simulink model "IDM_MOBIL"  (R2020a)
settings: Solver=VariableStepAuto  StartTime=0.0  StopTime=10.0  RelTol=1e-3
settings Model: Creator=Administrator  LastModifiedBy=Administrator

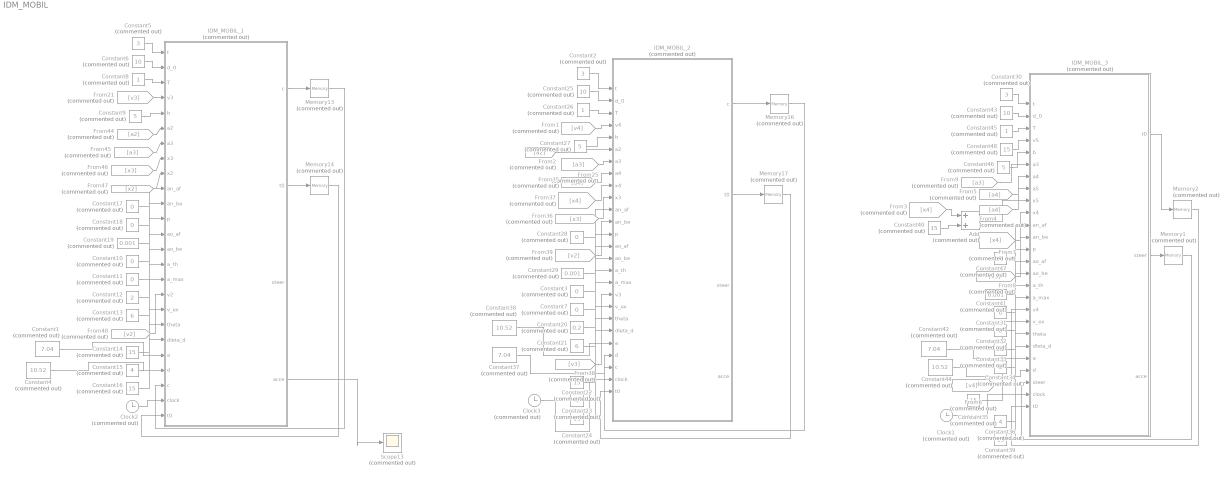
== system IDM_MOBIL ==
  Add : Sum  Commented=on
  Clock1 : Clock  Commented=on
  Clock2 : Clock  Commented=on
  Clock3 : Clock  Commented=on
  Constant1 : Constant  Commented=on  Value=7.04
  Constant{3,7,10..11,17..18,28,31..32,47} (10 alike) : Constant  Commented=on  Value=0
  Constant12 : Constant  Commented=on  Value=2
  Constant13 : Constant  Commented=on  Value=6
  Constant{14,16,22,24,35,39..40,48} (8 alike) : Constant  Commented=on  Value=15
  Constant15 : Constant  Commented=on  Value=4
  Constant19 : Constant  Commented=on  Value=0.001
  Constant2 : Constant  Commented=on  Value=3
  Constant20 : Constant  Commented=on  Value=0.2
  Constant21 : Constant  Commented=on  Value=6
  Constant23 : Constant  Commented=on  Value=4
  Constant25 : Constant  Commented=on  Value=10
  Constant26 : Constant  Commented=on
  Constant27 : Constant  Commented=on  Value=5
  Constant29 : Constant  Commented=on  Value=0.001
  Constant30 : Constant  Commented=on  Value=3
  Constant33 : Constant  Commented=on  Value=0.2
  Constant34 : Constant  Commented=on  Value=6
  Constant36 : Constant  Commented=on  Value=4
  Constant37 : Constant  Commented=on  Value=7.04
  Constant38 : Constant  Commented=on  Value=10.52
  Constant4 : Constant  Commented=on  Value=10.52
  Constant41 : Constant  Commented=on  Value=0.001
  Constant42 : Constant  Commented=on  Value=7.04
  Constant43 : Constant  Commented=on  Value=10
  Constant44 : Constant  Commented=on  Value=10.52
  Constant45 : Constant  Commented=on
  Constant46 : Constant  Commented=on  Value=5
  Constant5 : Constant  Commented=on  Value=3
  Constant6 : Constant  Commented=on  Value=10
  Constant8 : Constant  Commented=on
  Constant9 : Constant  Commented=on  Value=5
  From1 : From  Commented=on  GotoTag=v4  TagVisibility=global
  From2 : From  Commented=on  GotoTag=a2  TagVisibility=global
  From21 : From  Commented=on  GotoTag=v3  TagVisibility=global
  From25 : From  Commented=on  GotoTag=a3  TagVisibility=global
  From3 : From  Commented=on  GotoTag=x4  TagVisibility=global
  From35 : From  Commented=on  GotoTag=a4  TagVisibility=global
  From36 : From  Commented=on  GotoTag=x3  TagVisibility=global
  From37 : From  Commented=on  GotoTag=x4  TagVisibility=global
  From38 : From  Commented=on  GotoTag=v3  TagVisibility=global
  From39 : From  Commented=on  GotoTag=v2  TagVisibility=global
  From4 : From  Commented=on  GotoTag=a4  TagVisibility=global
  From44 : From  Commented=on  GotoTag=a2  TagVisibility=global
  From45 : From  Commented=on  GotoTag=a3  TagVisibility=global
  From46 : From  Commented=on  GotoTag=x3  TagVisibility=global
  From47 : From  Commented=on  GotoTag=x2  TagVisibility=global
  From48 : From  Commented=on  GotoTag=v2  TagVisibility=global
  From5 : From  Commented=on  GotoTag=a4  TagVisibility=global
  From6 : From  Commented=on  GotoTag=v4  TagVisibility=global
  From7 : From  Commented=on  GotoTag=x4  TagVisibility=global
  From8 : From  Commented=on  GotoTag=v3  TagVisibility=global
  From9 : From  Commented=on  GotoTag=a3  TagVisibility=global
  IDM_MOBIL_1 : MATLAB Function  Commented=on  TreatAsAtomicUnit=on
  IDM_MOBIL_2 : MATLAB Function  Commented=on  TreatAsAtomicUnit=on
  IDM_MOBIL_3 : MATLAB Function  Commented=on  TreatAsAtomicUnit=on
  Memory1 : Memory  Commented=on  InitialCondition=7.04
  Memory13 : Memory  Commented=on  InitialCondition=7.04
  Memory14 : Memory  Commented=on  InitialCondition=-3
  Memory16 : Memory  Commented=on  InitialCondition=10.52
  Memory17 : Memory  Commented=on  InitialCondition=-3
  Memory2 : Memory  Commented=on  InitialCondition=-3
  Scope13 : Scope  Commented=on
  wires:
  From48/1 -> IDM_MOBIL_1/17(v2)
  IDM_MOBIL_1/2(t0) -> Memory14/1
  Memory14/1 -> IDM_MOBIL_1/25("t0 ")
  Constant12/1 -> IDM_MOBIL_1/15(a_th)
  Memory13/1 -> IDM_MOBIL_1/23("c ")
  From47/1 -> IDM_MOBIL_1/9(x2)
  Constant15/1 -> IDM_MOBIL_1/19(theta)
  Constant10/1 -> IDM_MOBIL_1/13(ao_af)
  Constant16/1 -> IDM_MOBIL_1/20(dleta_d)
  Constant11/1 -> IDM_MOBIL_1/14(ao_be)
  Constant14/1 -> IDM_MOBIL_1/18(v_ex)
  From45/1 -> IDM_MOBIL_1/7(a3)
  Constant13/1 -> IDM_MOBIL_1/16(a_max)
  Constant5/1 -> IDM_MOBIL_1/1(t)
  From46/1 -> IDM_MOBIL_1/8(x3)
  Constant17/1 -> IDM_MOBIL_1/10(an_af)
  Constant19/1 -> IDM_MOBIL_1/12(p)
  Constant18/1 -> IDM_MOBIL_1/11(an_be)
  Clock2/1 -> IDM_MOBIL_1/24(clock)
  From44/1 -> IDM_MOBIL_1/6(a2)
  IDM_MOBIL_1/1(c) -> Memory13/1
  Constant4/1 -> IDM_MOBIL_1/22(d)
  Constant8/1 -> IDM_MOBIL_1/3(T)
  Constant1/1 -> IDM_MOBIL_1/21(a)
  IDM_MOBIL_1/4(acce) -> Scope13/1
  Constant6/1 -> IDM_MOBIL_1/2(d_0)
  From21/1 -> IDM_MOBIL_1/4(v3)
  Constant9/1 -> IDM_MOBIL_1/5(b)
  Constant21/1 -> IDM_MOBIL_2/17(a_max)
  Constant23/1 -> IDM_MOBIL_2/20(theta)
  Constant25/1 -> IDM_MOBIL_2/2(d_0)
  Constant24/1 -> IDM_MOBIL_2/21(dleta_d)
  Constant7/1 -> IDM_MOBIL_2/15(ao_be)
  IDM_MOBIL_2/1(c) -> Memory16/1
  IDM_MOBIL_2/2(t0) -> Memory17/1
  From2/1 -> IDM_MOBIL_2/6(a2)
  Constant37/1 -> IDM_MOBIL_2/23(d)
  Clock3/1 -> IDM_MOBIL_2/25(clock)
  Constant22/1 -> IDM_MOBIL_2/19(v_ex)
  Constant29/1 -> IDM_MOBIL_2/13(p)
  From38/1 -> IDM_MOBIL_2/18(v3)
  Memory17/1 -> IDM_MOBIL_2/26("t0 ")
  Constant20/1 -> IDM_MOBIL_2/16(a_th)
  Constant28/1 -> IDM_MOBIL_2/11(an_af)
  From25/1 -> IDM_MOBIL_2/7(a3)
  From37/1 -> IDM_MOBIL_2/9(x4)
  Constant3/1 -> IDM_MOBIL_2/14(ao_af)
  Constant38/1 -> IDM_MOBIL_2/22(a)
  Constant2/1 -> IDM_MOBIL_2/1(t)
  From39/1 -> IDM_MOBIL_2/12(an_be)
  From1/1 -> IDM_MOBIL_2/4(v4)
  Constant27/1 -> IDM_MOBIL_2/5(b)
  From36/1 -> IDM_MOBIL_2/10(x3)
  From35/1 -> IDM_MOBIL_2/8(a4)
  Constant26/1 -> IDM_MOBIL_2/3(T)
  Memory16/1 -> IDM_MOBIL_2/24("c ")
  IDM_MOBIL_3/1(t0) -> Memory2/1
  Constant47/1 -> IDM_MOBIL_3/11(an_af)
  Memory1/1 -> IDM_MOBIL_3/24("steer ")
  Constant36/1 -> IDM_MOBIL_3/20(theta)
  Memory2/1 -> IDM_MOBIL_3/26("t0 ")
  IDM_MOBIL_3/2(steer) -> Memory1/1
  From4/1 -> IDM_MOBIL_3/8(a5)
  Constant35/1 -> IDM_MOBIL_3/19(v_ex)
  Constant44/1 -> IDM_MOBIL_3/23(d)
  Constant34/1 -> IDM_MOBIL_3/17(a_max)
  Constant39/1 -> IDM_MOBIL_3/21(dleta_d)
  Constant31/1 -> IDM_MOBIL_3/14(ao_af)
  Constant42/1 -> IDM_MOBIL_3/22(a)
  From8/1 -> IDM_MOBIL_3/12(an_be)
  From6/1 -> IDM_MOBIL_3/18(v4)
  Constant46/1 -> IDM_MOBIL_3/5(b)
  From9/1 -> IDM_MOBIL_3/6(a3)
  From3/1 -> Add/1
  Constant48/1 -> IDM_MOBIL_3/4(v5)
  Constant30/1 -> IDM_MOBIL_3/1(t)
  From5/1 -> IDM_MOBIL_3/7(a4)
  Constant45/1 -> IDM_MOBIL_3/3(T)
  Constant32/1 -> IDM_MOBIL_3/15(ao_be)
  Clock1/1 -> IDM_MOBIL_3/25(clock)
  Constant43/1 -> IDM_MOBIL_3/2(d_0)
  Constant33/1 -> IDM_MOBIL_3/16(a_th)
  Constant41/1 -> IDM_MOBIL_3/13(p)
  From7/1 -> IDM_MOBIL_3/10(x4)
  Add/1 -> IDM_MOBIL_3/9(x5)
  Constant40/1 -> Add/2

== matlab function IDM_MOBIL/IDM_MOBIL_3 ==
  data: t0 output; t input; d_0 input; steer output; T input; v5 input; b input; a3 input; a4 input; a5 input; x5 input; x4 input; an_af input; an_be input; p input; ao_af input; ao_be input; a_th input; a_max input; v4 input; v_ex input; theta input; dleta_d input; acce output; a input; d input; steer input; clock input; t0 input
function [t0,steer,acce] = fcn(t,d_0,T,v5,b,a3,a4,a5,x5,x4,an_af,an_be,p,ao_af,ao_be,a_th,a_max,v4,v_ex,theta,dleta_d,a,d,steer,clock,t0)
delta_t = 3.5;
ac_be = a4;
vc_af = v4 + a4*t;
dleta_v = v5-v4;
dleta_cv_af = v5+a5*t-vc_af;
an_af = an_af+an_be+a3*t;
dleta_cd = x5+v5*t+0.5*a5*t^2-(x4+v4*t+0.5*a4*t^2);
dc_ex = d_0+T*vc_af+(vc_af*dleta_cv_af/(2*sqrt(a_max*b)));
ac_af = a_max*(1-(vc_af/v_ex)^theta-(dc_ex/dleta_cd)^2);
d_ex = d_0+T*v4+(v4*dleta_v/(2*sqrt(a_max*b)));
if clock-t0 > delta_t
    if ac_af-ac_be+p*(an_af-an_be+ao_af-ao_be) >= a_th
        if steer==a
            steer=d;
            acce = 0;
            t0=clock;
        else
            steer=a;
            acce = 0;
            t0=clock;
        end
    else
        steer=steer;
        acce = a_max*(1-(v4/v_ex)^theta-(d_ex/dleta_d)^2);
    end
else
    steer=steer;
    acce = 0;
    %acce = a_max*(1-(v4/v_ex)^theta-(d_ex/dleta_d)^2);
end

== matlab function IDM_MOBIL/IDM_MOBIL_1 ==
  data: c output; t0 output; t input; d_0 input; steer output; T input; v3 input; b input; a2 input; a3 input; x3 input; x2 input; an_af input; an_be input; p input; ao_af input; ao_be input; a_th input; a_max input; v2 input; v_ex input; theta input; dleta_d input; acce output; a input; d input; c input; clock input; t0 input
function [c,t0,steer,acce] = fcn(t,d_0,T,v3,b,a2,a3,x3,x2,an_af,an_be,p,ao_af,ao_be,a_th,a_max,v2,v_ex,theta,dleta_d,a,d,c,clock,t0)
delta_t = 3.5;
ac_be = a2;
vc_af = v2 + a2*t;
dleta_v = v3-v2;
dleta_cv_af = v3+a3*t-vc_af;
dleta_cd = x3+v3*t+0.5*a3*t^2-(x2+v2*t+0.5*a2*t^2);
dc_ex = d_0+T*vc_af+(vc_af*dleta_cv_af/(2*sqrt(a_max*b)));
ac_af = a_max*(1-(vc_af/v_ex)^theta-(dc_ex/dleta_cd)^2);
d_ex = d_0+T*v2+(v2*dleta_v/(2*sqrt(a_max*b)));
if clock-t0 > delta_t
    if ac_af-ac_be+p*(an_af-an_be+ao_af-ao_be) >= a_th
        if c==a
            c = d;
            steer=d;
            acce = 0;
            t0=clock;
        else
            c=a;
            steer=a;
            acce = 0;
            t0=clock;
        end
    else
        steer=c;
        acce = a_max*(1-(v2/v_ex)^theta-(d_ex/dleta_d)^2);
    end
else
    steer=c;
    acce = 0;
    %acce = a_max*(1-(v2/v_ex)^theta-(d_ex/dleta_d)^2);
end

== matlab function IDM_MOBIL/IDM_MOBIL_2 ==
  data: c output; t0 output; t input; d_0 input; steer output; T input; v4 input; b input; a2 input; a3 input; a4 input; x4 input; x3 input; an_af input; an_be input; p input; ao_af input; ao_be input; a_th input; a_max input; v3 input; v_ex input; theta input; dleta_d input; acce output; a input; d input; c input; clock input; t0 input
function [c,t0,steer,acce] = fcn(t,d_0,T,v4,b,a2,a3,a4,x4,x3,an_af,an_be,p,ao_af,ao_be,a_th,a_max,v3,v_ex,theta,dleta_d,a,d,c,clock,t0)
delta_t = 3.5;
ac_be = a3;
vc_af = v3 + a3*t;
dleta_v = v4-v3;
dleta_cv_af = v4+a4*t-vc_af;
an_af = an_af+an_be+a2*t;
dleta_cd = x4+v4*t+0.5*a4*t^2-(x3+v3*t+0.5*a3*t^2);
dc_ex = d_0+T*vc_af+(vc_af*dleta_cv_af/(2*sqrt(a_max*b)));
ac_af = a_max*(1-(vc_af/v_ex)^theta-(dc_ex/dleta_cd)^2);
d_ex = d_0+T*v3+(v3*dleta_v/(2*sqrt(a_max*b)));
if clock-t0 > delta_t
    if ac_af-ac_be+p*(an_af-an_be+ao_af-ao_be) >= a_th
        if c==a
            c = d;
            steer=d;
            acce = 0;
            t0=clock;
        else
            c=a;
            steer=a;
            acce = 0;
            t0=clock;
        end
    else
        steer=c;
        acce = a_max*(1-(v3/v_ex)^theta-(d_ex/dleta_d)^2);
    end
else
    steer=c;
    acce = 0;
    %acce = a_max*(1-(v3/v_ex)^theta-(d_ex/dleta_d)^2);
end
